simulink model "NetworkOrgignalparametrs3Copter"  (R2020a)
settings: Solver=FixedStepAuto  StartTime=0.0  StopTime=3  FixedStep=0.01  RelTol=1e-3
values from neighbouring files (symbols this model uses):
  Te = 0.012    [4двигателядообученный.mat]    (also in deepLearning.m; tdeepLearning.m)
  Tm = 0.025    [4двигателядообученный.mat]    (also in deepLearning.m; tdeepLearning.m)
  x1 = 1    [4двигателядообученный.mat]
  x2 = 1    [4двигателядообученный.mat]
  x3 = 1    [4двигателядообученный.mat]
libraries: dspsrcs4 x2, vrlib x1, rllib x1
settings Model: Creator=xreno  LastModifiedBy=xreno

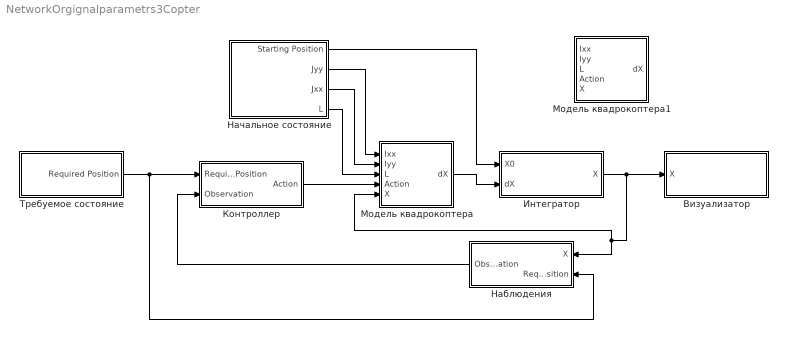
== system NetworkOrgignalparametrs3Copter ==
  Визуализатор : Subsystem
  Интегратор : Subsystem
  Контроллер : Subsystem
  Модель квадрокоптера : Subsystem
  Модель квадрокоптера1 : Subsystem
  Наблюдения : Subsystem
  Начальное состояние : Subsystem
  Требуемое состояние : Subsystem
  wires:
  Начальное состояние/2(Jyy) -> Модель квадрокоптера/1(Ixx)
  Начальное состояние/1(Starting Position) -> Интегратор/1(X0)
  Модель квадрокоптера/1(dX) -> Интегратор/2(dX)
  Требуемое состояние/1(Required Position) -> Наблюдения/2(Required Position), Контроллер/1(Required Position)
  Интегратор/1(X) -> Модель квадрокоптера/5(X), Наблюдения/1(X), Визуализатор/1(X)
  Начальное состояние/3(Jxx) -> Модель квадрокоптера/2(Iyy)
  Наблюдения/1(Observation) -> Контроллер/2(Observation)
  Начальное состояние/4(L) -> Модель квадрокоптера/3(L)
  Контроллер/1(Action) -> Модель квадрокоптера/4(Action)

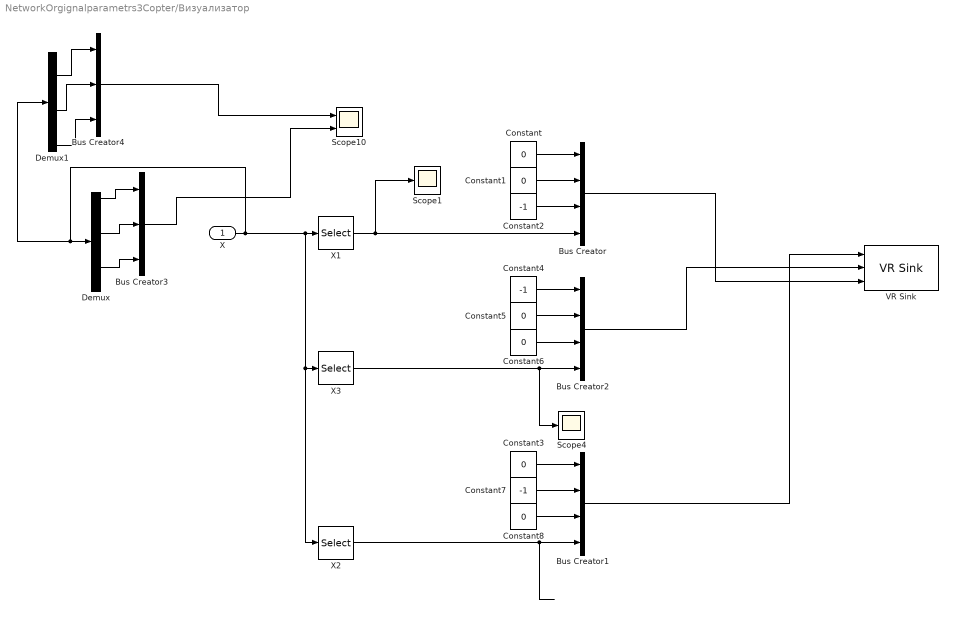
== system NetworkOrgignalparametrs3Copter/Визуализатор ==
  X : Inport
  Bus Creator : BusCreator  Inputs=4
  Bus Creator1 : BusCreator  Inputs=4
  Bus Creator2 : BusCreator  Inputs=4
  Bus Creator3 : BusCreator  Inputs=3
  Bus Creator4 : BusCreator  Inputs=3
  Constant{,1,3,5..6,8} (6 alike) : Constant  Value=0
  Constant2 : Constant  Value=-1
  Constant4 : Constant  Value=-1
  Constant7 : Constant  Value=-1
  Demux : Demux  Outputs=6
  Demux1 : Demux  Outputs=6
  Scope1 : Scope
  Scope10 : Scope  NumInputPorts=2
  Scope4 : Scope
  VR Sink : vrlib/VR Sink  InstantiateOnLoad=on  SampleTime=0.1  ViewEnable=on  RemoteChange=off  RemoteView=off  FieldsWritten=plane1.rotation.4.1.1.double#plane.rotation.4.1.1.double#quadro.rotation.4.1.1.double  WorldFileName=vrml1.wrl  AutoView=off  VideoDimensions=[200 320]  AllowVariableSize=off  FigureProperties="{'Position', 'Name', 'Viewpoint', 'CameraBound', 'CameraDirection', 'CameraPosition', 'CameraUpVector', 'ZoomFactor', 'Antialiasing', 'Headlight', 'Lighting', 'NavPanel', 'Sound', 'StatusBar', 'Stereo3D', 'Stereo3DCameraOffset', 'Stereo3DHIT', 'ToolBar', 'Textures', 'Transparency', 'Triad', 'Wireframe', 'NavZones', 'NavMode', 'NavSpeed', 'CaptureFileFormat', 'CaptureFileName', 'Record2DCompressMethod', 'Record2DCompressQuality', 'Record2D', 'Record2DFileName', 'Record2DFPS'; [1.0000000000000000e+00   7.4199999999999932e+01   1.5360000000000000e+03   6.9880000000000007e+02], '', '', 'on', [2.8420161502207653e-01  -9.0409149145346668e-01   3.1913636129464429e-01], [-2.2963536788759655e+00   7.6675017673078454e+00  -3.2677930566335149e+00], [6.8720478396535467e-01   4.2419952847847997e-01   5.8974939163497742e-01], [1.0000000000000000e+00], 'on', 'on', 'on', 'halfbar', 'on', 'on', 'off', [1.0000000149011612e-01], [0.0000000000000000e+00], 'on', 'on', 'on', 'none', 'off', 'off', 'examine', 'normal', 'tif', '%f_anim_%n.tif', 'auto', [7.5000000000000000e+01], 'on', '%f_anim_%n.avi', 'auto'}"
  X1 : Selector  InputPortWidth=6  IndexOptions=Index vector (dialog)  Indices=[1]  OutputSizes=1
  X2 : Selector  InputPortWidth=6  IndexOptions=Index vector (dialog)  Indices=[5]  OutputSizes=1
  X3 : Selector  InputPortWidth=6  IndexOptions=Index vector (dialog)  Indices=[3]  OutputSizes=1
  wires:
  Constant5/1 -> Bus Creator2/2
  Constant4/1 -> Bus Creator2/1
  Constant1/1 -> Bus Creator/2
  Bus Creator2/1 -> VR Sink/2
  Constant6/1 -> Bus Creator2/3
  Constant2/1 -> Bus Creator/3
  Constant/1 -> Bus Creator/1
  Bus Creator/1 -> VR Sink/3
  X1/1 -> Bus Creator/4, Scope1/1
  X3/1 -> Scope4/1, Bus Creator2/4
  Constant3/1 -> Bus Creator1/1
  X2/1 -> Bus Creator1/4
  Constant7/1 -> Bus Creator1/2
  Constant8/1 -> Bus Creator1/3
  Bus Creator1/1 -> VR Sink/1
  Demux/3 -> Bus Creator3/2
  Demux/5 -> Bus Creator3/3
  Demux/1 -> Bus Creator3/1
  Bus Creator3/1 -> Scope10/2
  X/1 -> Demux1/1, Demux/1, X2/1, X3/1, X1/1
  Demux1/2 -> Bus Creator4/1
  Demux1/4 -> Bus Creator4/2
  Demux1/6 -> Bus Creator4/3
  Bus Creator4/1 -> Scope10/1

== system NetworkOrgignalparametrs3Copter/Интегратор ==
  X0 : Inport
  dX : Inport  Port=2
  Integrator2 : Integrator  InitialConditionSource=external
  X : Outport
  wires:
  X0/1 -> Integrator2/2
  dX/1 -> Integrator2/1
  Integrator2/1 -> X/1

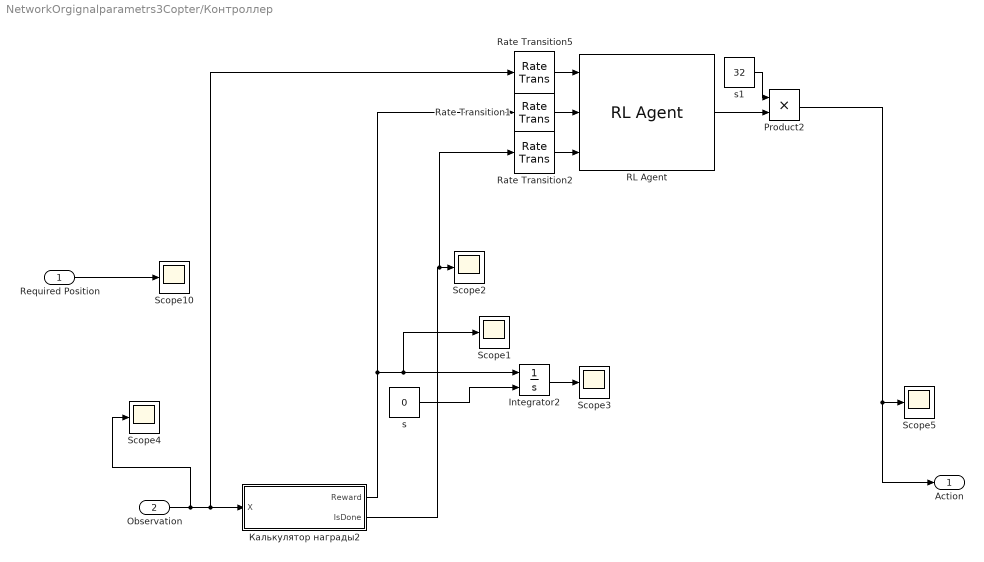
== system NetworkOrgignalparametrs3Copter/Контроллер ==
  Required Position : Inport
  Observation : Inport  Port=2
  Integrator2 : Integrator  InitialConditionSource=external
  Product2 : Product
  RL Agent : rllib/RL Agent  Agent=agent  ProvideReward=on  ProvideIsDone=on  ProvideCumRwd=off  TreatAsDirectFeedthrough=on  CollectLoggedSignals=on  CollectModelStates=on
  Rate Transition1 : RateTransition
  Rate Transition2 : RateTransition
  Rate Transition5 : RateTransition
  Scope{1..5,10} (6 alike) : Scope
  s : Constant  Value=0
  s1 : Constant  Value=32
  Калькулятор награды2 : Subsystem
  Action : Outport
  wires:
  Required Position/1 -> Scope10/1
  Integrator2/1 -> Scope3/1
  s/1 -> Integrator2/2
  Калькулятор награды2/1(Reward) -> Rate Transition1/1, Scope1/1, Integrator2/1
  Калькулятор награды2/2(IsDone) -> Rate Transition2/1, Scope2/1
  Product2/1 -> Action/1, Scope5/1
  Observation/1 -> Scope4/1, Rate Transition5/1, Калькулятор награды2/1(X)
  RL Agent/1 -> Product2/2
  s1/1 -> Product2/1
  Rate Transition5/1 -> RL Agent/1
  Rate Transition1/1 -> RL Agent/2
  Rate Transition2/1 -> RL Agent/3

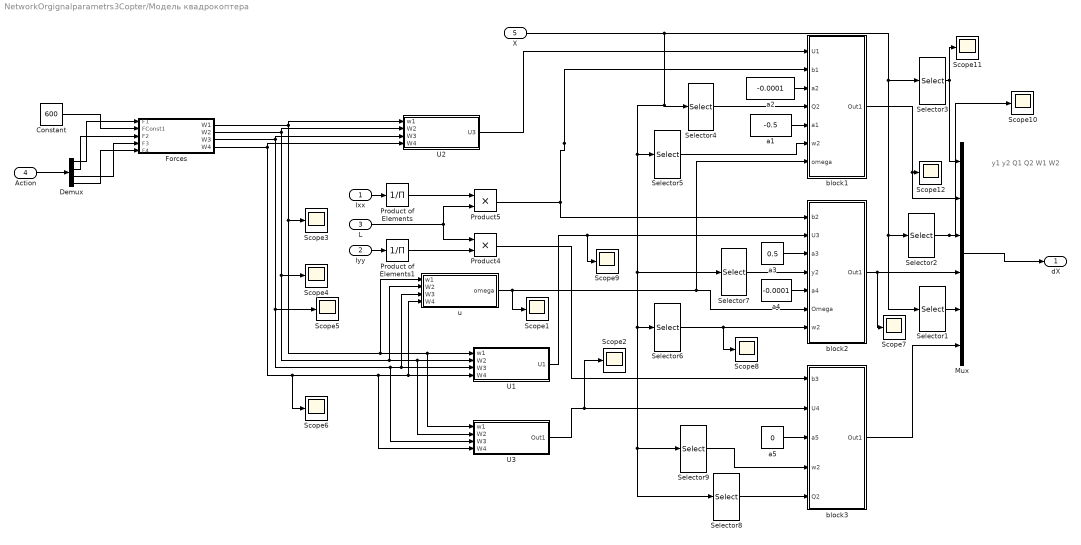
== system NetworkOrgignalparametrs3Copter/Модель квадрокоптера ==
  note: y1
      | y2
      | Q1
      | Q2
      | W1
      | W2
  Ixx : Inport
  Iyy : Inport  Port=2
  L : Inport  Port=3
  Action : Inport  Port=4
  X : Inport  Port=5
  Constant : Constant  Value=600
  Demux : Demux
  Forces : Subsystem
  Mux : Mux  Inputs=6
  Product of Elements : Product  Inputs=/
  Product of Elements1 : Product  Inputs=/
  Product4 : Product
  Product5 : Product
  Scope{1..12} (12 alike) : Scope
  Selector{1,5..6,9} (4 alike) : Selector  InputPortWidth=6  IndexOptions=Index vector (dialog)  Indices=[6]  OutputSizes=1
  Selector2 : Selector  InputPortWidth=6  IndexOptions=Index vector (dialog)  Indices=[4]  OutputSizes=1
  Selector3 : Selector  InputPortWidth=6  IndexOptions=Index vector (dialog)  Indices=[2]  OutputSizes=1
  Selector4 : Selector  InputPortWidth=6  IndexOptions=Index vector (dialog)  Indices=[4]  OutputSizes=1
  Selector7 : Selector  InputPortWidth=6  IndexOptions=Index vector (dialog)  Indices=[2]  OutputSizes=1
  Selector8 : Selector  InputPortWidth=6  IndexOptions=Index vector (dialog)  Indices=[4]  OutputSizes=1
  U1 : Subsystem
  U2 : Subsystem
  U3 : Subsystem
  a1 : Constant  Value=-0.5
  a2 : Constant  Value=-0.0001
  a3 : Constant  Value=0.5
  a4 : Constant  Value=-0.0001
  a5 : Constant  Value=0
  block1 : Subsystem
  block2 : Subsystem
  block3 : Subsystem
  u : Subsystem
  dX : Outport
  wires:
  X/1 -> Selector7/1, Selector8/1, Selector9/1, Selector6/1, Selector5/1, Selector4/1, Selector1/1, Selector2/1, Selector3/1
  Action/1 -> Demux/1
  Mux/1 -> dX/1
  Forces/2(W2) -> U2/2(W2), Scope4/1, u/2(W2), U1/2(W2), U3/2(W2)
  Forces/4(W4) -> U2/4(W4), Scope6/1, U3/4(W4), u/4(W4), U1/4(W4)
  Forces/3(W3) -> U2/3(W3), U3/3(W3), u/3(W3), U1/3(W3), Scope5/1
  U2/1(U3) -> block1/1(U1)
  Product5/1 -> block1/2(b1), block2/1(b2)
  U1/1(U1) -> Scope9/1, block2/2(U3)
  Product of Elements/1 -> Product5/1
  Product of Elements1/1 -> Product4/2
  Product4/1 -> block3/1(b3)
  L/1 -> Product4/1, Product5/2
  Iyy/1 -> Product of Elements1/1
  Ixx/1 -> Product of Elements/1
  Forces/1(W1) -> U2/1(w1), u/1(w1), U1/1(w1), U3/1(w1), Scope3/1
  block1/1(Out1) -> Scope12/1, Mux/2
  block2/1(Out1) -> Scope7/1, Mux/4
  block3/1(Out1) -> Mux/6
  Selector3/1 -> Scope11/1, Mux/1
  Selector2/1 -> Scope10/1, Mux/3
  Selector1/1 -> Mux/5
  u/1(omega) -> Scope1/1, block2/6(Omega), block1/7(omega)
  a3/1 -> block2/3(a3)
  a1/1 -> block1/5(a1)
  a2/1 -> block1/3(a2)
  a4/1 -> block2/5(a4)
  a5/1 -> block3/3(a5)
  U3/1(Out1) -> Scope2/1, block3/2(U4)
  Selector4/1 -> block1/4(Q2)
  Selector5/1 -> block1/6(w2)
  Selector6/1 -> Scope8/1, block2/7(w2)
  Selector7/1 -> block2/4(y2)
  Selector8/1 -> block3/5(Q2)
  Selector9/1 -> block3/4(w2)
  Demux/1 -> Forces/1(F1)
  Constant/1 -> Forces/2(FConst1)
  Demux/2 -> Forces/3(F2)
  Demux/3 -> Forces/4(F3)
  Demux/4 -> Forces/5(F4)

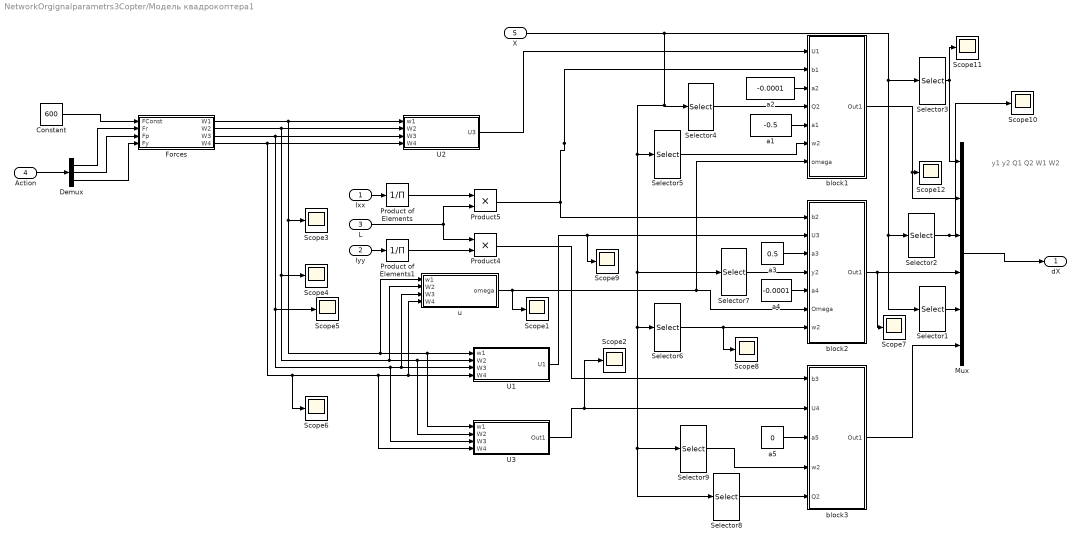
== system NetworkOrgignalparametrs3Copter/Модель квадрокоптера1 ==
  note: y1
      | y2
      | Q1
      | Q2
      | W1
      | W2
  Ixx : Inport
  Iyy : Inport  Port=2
  L : Inport  Port=3
  Action : Inport  Port=4
  X : Inport  Port=5
  Constant : Constant  Value=600
  Demux : Demux  Outputs=3
  Forces : Subsystem
  Mux : Mux  Inputs=6
  Product of Elements : Product  Inputs=/
  Product of Elements1 : Product  Inputs=/
  Product4 : Product
  Product5 : Product
  Scope{1..12} (12 alike) : Scope
  Selector{1,5..6,9} (4 alike) : Selector  InputPortWidth=6  IndexOptions=Index vector (dialog)  Indices=[6]  OutputSizes=1
  Selector2 : Selector  InputPortWidth=6  IndexOptions=Index vector (dialog)  Indices=[4]  OutputSizes=1
  Selector3 : Selector  InputPortWidth=6  IndexOptions=Index vector (dialog)  Indices=[2]  OutputSizes=1
  Selector4 : Selector  InputPortWidth=6  IndexOptions=Index vector (dialog)  Indices=[4]  OutputSizes=1
  Selector7 : Selector  InputPortWidth=6  IndexOptions=Index vector (dialog)  Indices=[2]  OutputSizes=1
  Selector8 : Selector  InputPortWidth=6  IndexOptions=Index vector (dialog)  Indices=[4]  OutputSizes=1
  U1 : Subsystem
  U2 : Subsystem
  U3 : Subsystem
  a1 : Constant  Value=-0.5
  a2 : Constant  Value=-0.0001
  a3 : Constant  Value=0.5
  a4 : Constant  Value=-0.0001
  a5 : Constant  Value=0
  block1 : Subsystem
  block2 : Subsystem
  block3 : Subsystem
  u : Subsystem
  dX : Outport
  wires:
  X/1 -> Selector7/1, Selector8/1, Selector9/1, Selector6/1, Selector5/1, Selector4/1, Selector1/1, Selector2/1, Selector3/1
  Action/1 -> Demux/1
  Mux/1 -> dX/1
  Constant/1 -> Forces/1(FConst)
  Forces/2(W2) -> U2/2(W2), Scope4/1, u/2(W2), U1/2(W2), U3/2(W2)
  Forces/4(W4) -> U2/4(W4), Scope6/1, U3/4(W4), u/4(W4), U1/4(W4)
  Forces/3(W3) -> U2/3(W3), U3/3(W3), u/3(W3), U1/3(W3), Scope5/1
  U2/1(U3) -> block1/1(U1)
  Product5/1 -> block1/2(b1), block2/1(b2)
  U1/1(U1) -> Scope9/1, block2/2(U3)
  Product of Elements/1 -> Product5/1
  Product of Elements1/1 -> Product4/2
  Product4/1 -> block3/1(b3)
  L/1 -> Product4/1, Product5/2
  Iyy/1 -> Product of Elements1/1
  Ixx/1 -> Product of Elements/1
  Forces/1(W1) -> U2/1(w1), u/1(w1), U1/1(w1), U3/1(w1), Scope3/1
  Demux/1 -> Forces/2(Fr)
  Demux/2 -> Forces/3(Fp)
  block1/1(Out1) -> Scope12/1, Mux/2
  block2/1(Out1) -> Scope7/1, Mux/4
  block3/1(Out1) -> Mux/6
  Selector3/1 -> Scope11/1, Mux/1
  Selector2/1 -> Scope10/1, Mux/3
  Selector1/1 -> Mux/5
  u/1(omega) -> Scope1/1, block2/6(Omega), block1/7(omega)
  a3/1 -> block2/3(a3)
  a1/1 -> block1/5(a1)
  a2/1 -> block1/3(a2)
  a4/1 -> block2/5(a4)
  a5/1 -> block3/3(a5)
  U3/1(Out1) -> Scope2/1, block3/2(U4)
  Selector4/1 -> block1/4(Q2)
  Selector5/1 -> block1/6(w2)
  Selector6/1 -> Scope8/1, block2/7(w2)
  Selector7/1 -> block2/4(y2)
  Selector8/1 -> block3/5(Q2)
  Selector9/1 -> block3/4(w2)
  Demux/3 -> Forces/4(Fy)

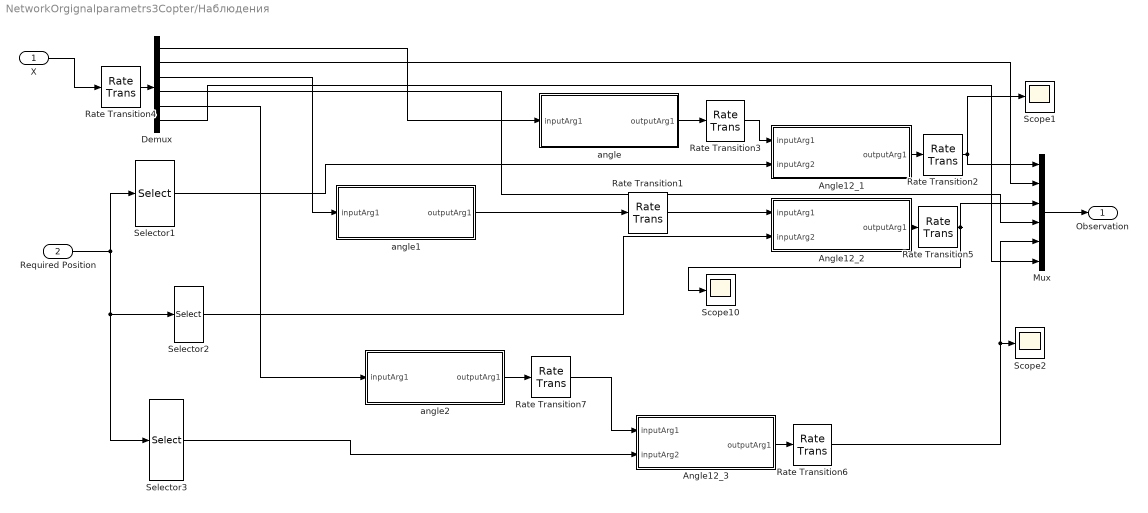
== system NetworkOrgignalparametrs3Copter/Наблюдения ==
  X : Inport
  Required Position : Inport  Port=2
  Angle12_1 : MATLAB Function  TreatAsAtomicUnit=on
  Angle12_2 : MATLAB Function  TreatAsAtomicUnit=on
  Angle12_3 : MATLAB Function  TreatAsAtomicUnit=on
  Demux : Demux  Outputs=6
  Mux : Mux  Inputs=6
  Rate Transition{1..7} (7 alike) : RateTransition
  Scope1 : Scope
  Scope10 : Scope
  Scope2 : Scope
  Selector1 : Selector  InputPortWidth=6  IndexOptions=Index vector (dialog)  Indices=[1]  OutputSizes=1
  Selector2 : Selector  InputPortWidth=6  IndexOptions=Index vector (dialog)  Indices=[3]  OutputSizes=1
  Selector3 : Selector  InputPortWidth=6  IndexOptions=Index vector (dialog)  Indices=[5]  OutputSizes=1
  angle : MATLAB Function  TreatAsAtomicUnit=on
  angle1 : MATLAB Function  TreatAsAtomicUnit=on
  angle2 : MATLAB Function  TreatAsAtomicUnit=on
  Observation : Outport
  wires:
  Rate Transition5/1 -> Scope10/1, Mux/3
  Rate Transition2/1 -> Mux/1, Scope1/1
  Mux/1 -> Observation/1
  Required Position/1 -> Selector1/1, Selector3/1, Selector2/1
  Selector1/1 -> Angle12_1/2(inputArg2)
  Demux/3 -> angle1/1(inputArg1)
  angle1/1(outputArg1) -> Rate Transition1/1
  Rate Transition3/1 -> Angle12_1/1(inputArg1)
  Demux/2 -> Mux/2
  Demux/4 -> Mux/4
  Selector2/1 -> Angle12_2/2(inputArg2)
  X/1 -> Rate Transition4/1
  Rate Transition6/1 -> Scope2/1, Mux/5
  Rate Transition7/1 -> Angle12_3/1(inputArg1)
  Selector3/1 -> Angle12_3/2(inputArg2)
  Demux/5 -> angle2/1(inputArg1)
  Demux/6 -> Mux/6
  angle/1(outputArg1) -> Rate Transition3/1
  Demux/1 -> angle/1(inputArg1)
  Angle12_1/1(outputArg1) -> Rate Transition2/1
  Rate Transition4/1 -> Demux/1
  Rate Transition1/1 -> Angle12_2/1(inputArg1)
  Angle12_2/1(outputArg1) -> Rate Transition5/1
  Angle12_3/1(outputArg1) -> Rate Transition6/1
  angle2/1(outputArg1) -> Rate Transition7/1

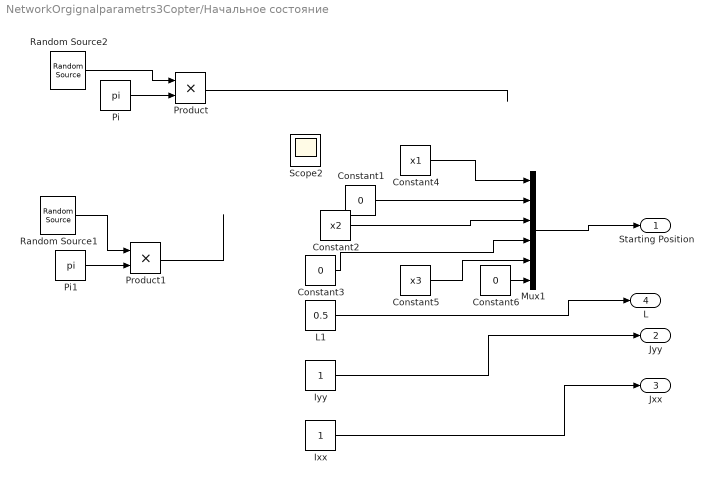
== system NetworkOrgignalparametrs3Copter/Начальное состояние ==
  Constant1 : Constant  Value=0
  Constant2 : Constant  Value=x2
  Constant3 : Constant  Value=0
  Constant4 : Constant  Value=x1
  Constant5 : Constant  Value=x3
  Constant6 : Constant  Value=0
  Ixx : Constant
  Iyy : Constant
  L1 : Constant  Value=0.5
  Mux1 : Mux  Inputs=6
  Pi : Constant  Value=pi  OutDataTypeStr=Inherit: Inherit via back propagation
  Pi1 : Constant  Value=pi  OutDataTypeStr=Inherit: Inherit via back propagation
  Product : Product
  Product1 : Product
  Random Source1 : dspsrcs4/Random Source  SrcType=Uniform  NormMethod=Ziggurat  CltLength=12  MinVal=-1  MaxVal=1  MeanVal=0  VarVal=1  RepMode=Not repeatable  rawSeed=1  IsInherit=off  SampMode=Discrete  SampTime=1  SampFrame=1  DataType=Double  OutComplex=Real  OutputFrames=off
  Random Source2 : dspsrcs4/Random Source  SrcType=Uniform  NormMethod=Ziggurat  CltLength=12  MinVal=-1  MaxVal=1  MeanVal=0  VarVal=1  RepMode=Not repeatable  rawSeed=1  IsInherit=off  SampMode=Discrete  SampTime=1  SampFrame=1  DataType=Double  OutComplex=Real  OutputFrames=off
  Scope2 : Scope
  Starting Position : Outport
  Jyy : Outport  Port=2
  Jxx : Outport  Port=3
  L : Outport  Port=4
  wires:
  Constant1/1 -> Mux1/2
  Mux1/1 -> Starting Position/1
  Constant3/1 -> Mux1/4
  Ixx/1 -> Jxx/1
  Iyy/1 -> Jyy/1
  L1/1 -> L/1
  Pi/1 -> Product/2
  Random Source2/1 -> Product/1
  Random Source1/1 -> Product1/1
  Pi1/1 -> Product1/2
  Product1/1 -> ?
  Product/1 -> ?
  Constant2/1 -> Mux1/3
  Constant4/1 -> Mux1/1
  Constant5/1 -> Mux1/5
  Constant6/1 -> Mux1/6

== system NetworkOrgignalparametrs3Copter/Требуемое состояние ==
  Constant{,1..5} (6 alike) : Constant  Value=0
  Mux1 : Mux  Inputs=6
  Required Position : Outport
  wires:
  Constant/1 -> Mux1/1
  Constant3/1 -> Mux1/4
  Constant1/1 -> Mux1/2
  Mux1/1 -> Required Position/1
  Constant2/1 -> Mux1/3
  Constant4/1 -> Mux1/5
  Constant5/1 -> Mux1/6

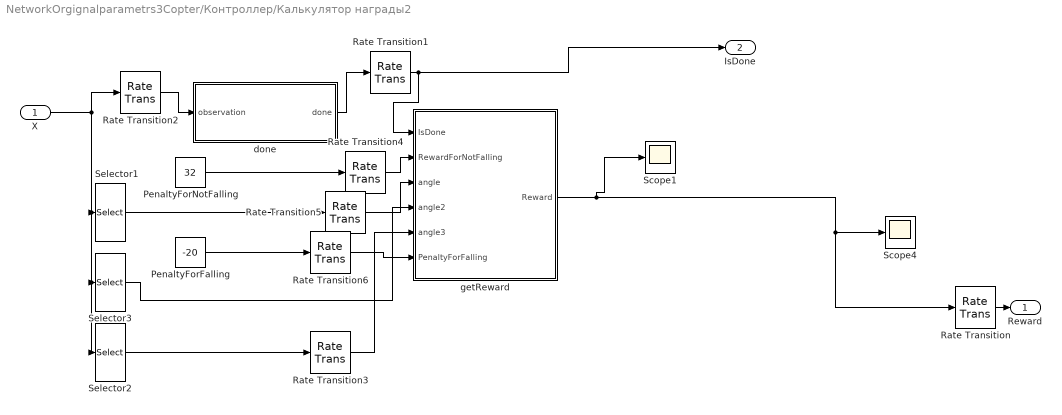
== system NetworkOrgignalparametrs3Copter/Контроллер/Калькулятор награды2 ==
  X : Inport
  PenaltyForFalling : Constant  Value=-20
  PenaltyForNotFalling : Constant  Value=32
  Rate Transition{,1..6} (7 alike) : RateTransition
  Scope1 : Scope
  Scope4 : Scope
  Selector1 : Selector  InputPortWidth=6  IndexOptions=Index vector (dialog)  Indices=[1]  OutputSizes=1
  Selector2 : Selector  InputPortWidth=6  IndexOptions=Index vector (dialog)  Indices=[5]  OutputSizes=1
  Selector3 : Selector  InputPortWidth=6  IndexOptions=Index vector (dialog)  Indices=[3]  OutputSizes=1
  done : MATLAB Function  TreatAsAtomicUnit=on
  getReward : MATLAB Function  TreatAsAtomicUnit=on
  Reward : Outport
  IsDone : Outport  Port=2
  wires:
  X/1 -> Rate Transition2/1, Selector2/1, Selector3/1, Selector1/1
  done/1(done) -> Rate Transition1/1
  PenaltyForFalling/1 -> Rate Transition6/1
  PenaltyForNotFalling/1 -> Rate Transition4/1
  Selector1/1 -> Rate Transition5/1
  getReward/1(Reward) -> Scope4/1, Rate Transition/1, Scope1/1
  Rate Transition/1 -> Reward/1
  Rate Transition2/1 -> done/1(observation)
  Rate Transition1/1 -> getReward/1(IsDone), IsDone/1
  Rate Transition4/1 -> getReward/2(RewardForNotFalling)
  Rate Transition5/1 -> getReward/3(angle)
  Rate Transition6/1 -> getReward/6(PenaltyForFalling)
  Selector3/1 -> getReward/4(angle2)
  Selector2/1 -> Rate Transition3/1
  Rate Transition3/1 -> getReward/5(angle3)

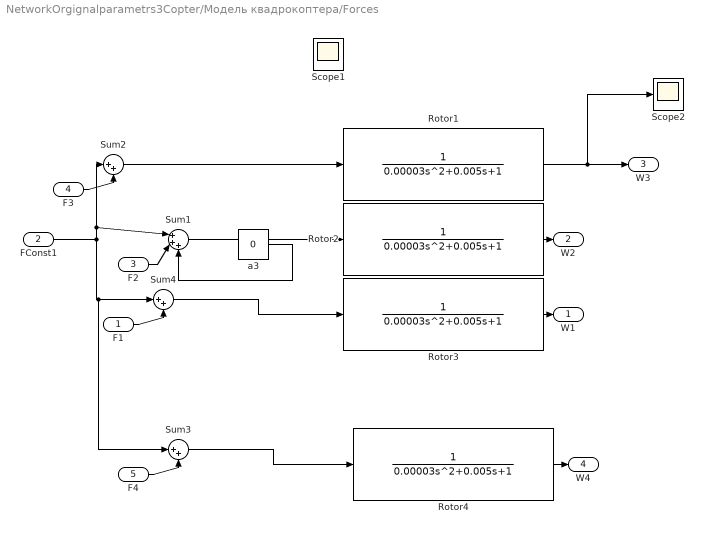
== system NetworkOrgignalparametrs3Copter/Модель квадрокоптера/Forces ==
  F1 : Inport
  FConst1 : Inport  Port=2
  F2 : Inport  Port=3
  F3 : Inport  Port=4
  F4 : Inport  Port=5
  Rotor{1..4} (4 alike) : TransferFcn  Denominator=[0.00003 0.005 1]
  Scope1 : Scope
  Scope2 : Scope
  Sum1 : Sum  Inputs=|+++
  Sum2 : Sum  Inputs=|++
  Sum3 : Sum  Inputs=|++
  Sum4 : Sum  Inputs=|++
  a3 : Constant  Value=0
  W1 : Outport
  W2 : Outport  Port=2
  W3 : Outport  Port=3
  W4 : Outport  Port=4
  wires:
  Rotor1/1 -> Scope2/1, W3/1
  Rotor2/1 -> W2/1
  Rotor3/1 -> W1/1
  Rotor4/1 -> W4/1
  Sum4/1 -> Rotor3/1
  F1/1 -> Sum4/2
  F2/1 -> Sum1/2
  Sum1/1 -> Rotor2/1
  F3/1 -> Sum2/2
  Sum2/1 -> Rotor1/1
  Sum3/1 -> Rotor4/1
  FConst1/1 -> Sum2/1, Sum1/1, Sum3/1, Sum4/1
  F4/1 -> Sum3/2
  a3/1 -> Sum1/3

== system NetworkOrgignalparametrs3Copter/Модель квадрокоптера/U1 ==
  w1 : Inport
  W2 : Inport  Port=2
  W3 : Inport  Port=3
  W4 : Inport  Port=4
  Add : Sum  Inputs=++--
  Product{,1..4} (5 alike) : Product
  b : Constant  Value=0.001
  U1 : Outport
  wires:
  Add/1 -> Product4/2
  W4/1 -> Product3/2, Product3/1
  Product2/1 -> Add/3
  Product/1 -> Add/1
  w1/1 -> Product/2, Product/1
  Product1/1 -> Add/2
  W2/1 -> Product1/2, Product1/1
  W3/1 -> Product2/2, Product2/1
  Product3/1 -> Add/4
  b/1 -> Product4/1
  Product4/1 -> U1/1

== system NetworkOrgignalparametrs3Copter/Модель квадрокоптера/U2 ==
  w1 : Inport
  W2 : Inport  Port=2
  W3 : Inport  Port=3
  W4 : Inport  Port=4
  Add : Sum  Inputs=+-+-
  Product{,1..4} (5 alike) : Product
  b : Constant  Value=0.001
  U3 : Outport
  wires:
  w1/1 -> Product/2, Product/1
  W2/1 -> Product1/2, Product1/1
  W3/1 -> Product2/2, Product2/1
  W4/1 -> Product3/2, Product3/1
  Product/1 -> Add/1
  Product1/1 -> Add/2
  Product2/1 -> Add/3
  Product3/1 -> Add/4
  b/1 -> Product4/1
  Add/1 -> Product4/2
  Product4/1 -> U3/1

== system NetworkOrgignalparametrs3Copter/Модель квадрокоптера/U3 ==
  w1 : Inport
  W2 : Inport  Port=2
  W3 : Inport  Port=3
  W4 : Inport  Port=4
  Add : Sum  Inputs=-++-
  Product{,1..4} (5 alike) : Product
  b1 : Constant  Value=0.0008
  Out1 : Outport
  wires:
  Add/1 -> Product4/2
  W4/1 -> Product3/2, Product3/1
  Product2/1 -> Add/3
  Product/1 -> Add/1
  w1/1 -> Product/2, Product/1
  Product1/1 -> Add/2
  W2/1 -> Product1/2, Product1/1
  W3/1 -> Product2/2, Product2/1
  Product3/1 -> Add/4
  b1/1 -> Product4/1
  Product4/1 -> Out1/1

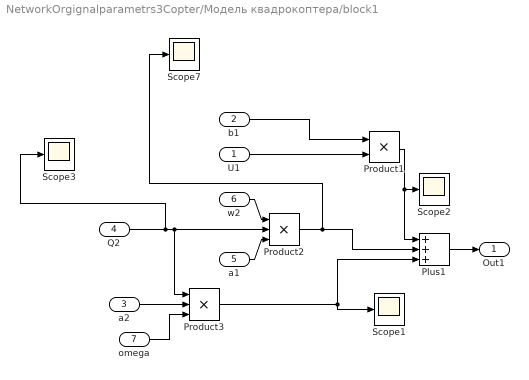
== system NetworkOrgignalparametrs3Copter/Модель квадрокоптера/block1 ==
  U1 : Inport
  b1 : Inport  Port=2
  a2 : Inport  Port=3
  Q2 : Inport  Port=4
  a1 : Inport  Port=5
  w2 : Inport  Port=6
  omega : Inport  Port=7
  Plus1 : Sum  Inputs=+++
  Product1 : Product
  Product2 : Product  Inputs=3
  Product3 : Product  Inputs=3
  Scope{1..3,7} (4 alike) : Scope
  Out1 : Outport
  wires:
  b1/1 -> Product1/1
  U1/1 -> Product1/2
  w2/1 -> Product2/1
  a1/1 -> Product2/3
  Q2/1 -> Scope3/1, Product3/1, Product2/2
  a2/1 -> Product3/2
  omega/1 -> Product3/3
  Product1/1 -> Scope2/1, Plus1/1
  Product2/1 -> Scope7/1, Plus1/2
  Product3/1 -> Plus1/3, Scope1/1
  Plus1/1 -> Out1/1

== system NetworkOrgignalparametrs3Copter/Модель квадрокоптера/block2 ==
  b2 : Inport
  U3 : Inport  Port=2
  a3 : Inport  Port=3
  y2 : Inport  Port=4
  a4 : Inport  Port=5
  Omega : Inport  Port=6
  w2 : Inport  Port=7
  Plus1 : Sum  Inputs=+++
  Product1 : Product
  Product2 : Product  Inputs=3
  Product3 : Product  Inputs=3
  Out1 : Outport
  wires:
  b2/1 -> Product1/1
  U3/1 -> Product1/2
  Omega/1 -> Product2/1
  a4/1 -> Product2/3
  y2/1 -> Product3/1, Product2/2
  a3/1 -> Product3/2
  w2/1 -> Product3/3
  Product1/1 -> Plus1/1
  Product2/1 -> Plus1/2
  Product3/1 -> Plus1/3
  Plus1/1 -> Out1/1

== system NetworkOrgignalparametrs3Copter/Модель квадрокоптера/block3 ==
  b3 : Inport
  U4 : Inport  Port=2
  a5 : Inport  Port=3
  w2 : Inport  Port=4
  Q2 : Inport  Port=5
  Plus1 : Sum  Inputs=-+
  Product1 : Product
  Product3 : Product  Inputs=3
  Out1 : Outport
  wires:
  b3/1 -> Product1/1
  U4/1 -> Product1/2
  a5/1 -> Product3/2
  Product1/1 -> Plus1/1
  Product3/1 -> Plus1/2
  Plus1/1 -> Out1/1
  w2/1 -> Product3/3
  Q2/1 -> Product3/1

== system NetworkOrgignalparametrs3Copter/Модель квадрокоптера/u ==
  w1 : Inport
  W2 : Inport  Port=2
  W3 : Inport  Port=3
  W4 : Inport  Port=4
  Add : Sum  Inputs=+--+
  omega : Outport
  wires:
  w1/1 -> Add/1
  W2/1 -> Add/2
  W3/1 -> Add/3
  W4/1 -> Add/4
  Add/1 -> omega/1

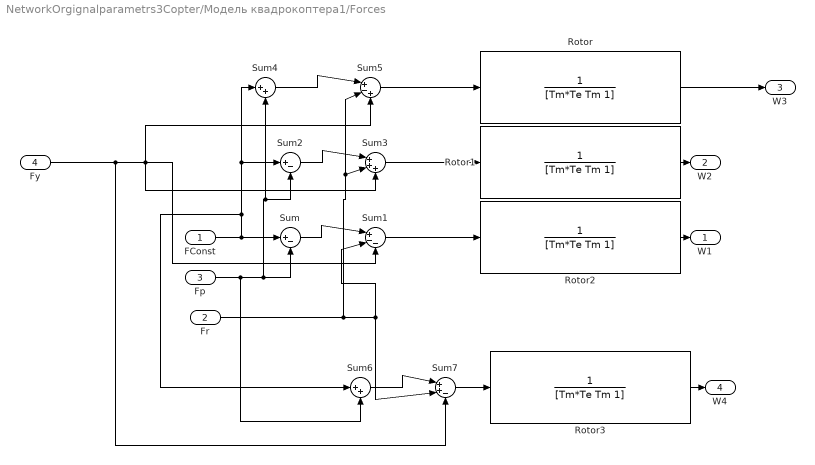
== system NetworkOrgignalparametrs3Copter/Модель квадрокоптера1/Forces ==
  FConst : Inport
  Fr : Inport  Port=2
  Fp : Inport  Port=3
  Fy : Inport  Port=4
  Rotor{,1..3} (4 alike) : TransferFcn  Denominator=[Tm*Te Tm 1]
  Sum : Sum  Inputs=|+-
  Sum1 : Sum  Inputs=|+--
  Sum2 : Sum  Inputs=|+-
  Sum3 : Sum  Inputs=|+++
  Sum4 : Sum  Inputs=|++
  Sum5 : Sum  Inputs=|+-+
  Sum6 : Sum  Inputs=|++
  Sum7 : Sum  Inputs=|++-
  W1 : Outport
  W2 : Outport  Port=2
  W3 : Outport  Port=3
  W4 : Outport  Port=4
  wires:
  Sum/1 -> Sum1/1
  Fp/1 -> Sum6/2, Sum4/2, Sum2/2, Sum/2
  Fr/1 -> Sum3/2, Sum5/2, Sum1/2, Sum7/2
  Sum2/1 -> Sum3/1
  Sum4/1 -> Sum5/1
  Sum6/1 -> Sum7/1
  FConst/1 -> Sum6/1, Sum4/1, Sum2/1, Sum/1
  Sum5/1 -> Rotor/1
  Sum7/1 -> Rotor3/1
  Sum1/1 -> Rotor2/1
  Sum3/1 -> Rotor1/1
  Fy/1 -> Sum1/3, Sum3/3, Sum5/3, Sum7/3
  Rotor/1 -> W3/1
  Rotor1/1 -> W2/1
  Rotor2/1 -> W1/1
  Rotor3/1 -> W4/1

== system NetworkOrgignalparametrs3Copter/Модель квадрокоптера1/U1 ==
  w1 : Inport
  W2 : Inport  Port=2
  W3 : Inport  Port=3
  W4 : Inport  Port=4
  Add : Sum  Inputs=++--
  Product{,1..4} (5 alike) : Product
  b : Constant  Value=0.001
  U1 : Outport
  wires:
  Add/1 -> Product4/2
  W4/1 -> Product3/2, Product3/1
  Product2/1 -> Add/3
  Product/1 -> Add/1
  w1/1 -> Product/2, Product/1
  Product1/1 -> Add/2
  W2/1 -> Product1/2, Product1/1
  W3/1 -> Product2/2, Product2/1
  Product3/1 -> Add/4
  b/1 -> Product4/1
  Product4/1 -> U1/1

== system NetworkOrgignalparametrs3Copter/Модель квадрокоптера1/U2 ==
  w1 : Inport
  W2 : Inport  Port=2
  W3 : Inport  Port=3
  W4 : Inport  Port=4
  Add : Sum  Inputs=+-+-
  Product{,1..4} (5 alike) : Product
  b : Constant  Value=0.001
  U3 : Outport
  wires:
  w1/1 -> Product/2, Product/1
  W2/1 -> Product1/2, Product1/1
  W3/1 -> Product2/2, Product2/1
  W4/1 -> Product3/2, Product3/1
  Product/1 -> Add/1
  Product1/1 -> Add/2
  Product2/1 -> Add/3
  Product3/1 -> Add/4
  b/1 -> Product4/1
  Add/1 -> Product4/2
  Product4/1 -> U3/1

== system NetworkOrgignalparametrs3Copter/Модель квадрокоптера1/U3 ==
  w1 : Inport
  W2 : Inport  Port=2
  W3 : Inport  Port=3
  W4 : Inport  Port=4
  Add : Sum  Inputs=-++-
  Product{,1..4} (5 alike) : Product
  b1 : Constant  Value=0.0008
  Out1 : Outport
  wires:
  Add/1 -> Product4/2
  W4/1 -> Product3/2, Product3/1
  Product2/1 -> Add/3
  Product/1 -> Add/1
  w1/1 -> Product/2, Product/1
  Product1/1 -> Add/2
  W2/1 -> Product1/2, Product1/1
  W3/1 -> Product2/2, Product2/1
  Product3/1 -> Add/4
  b1/1 -> Product4/1
  Product4/1 -> Out1/1

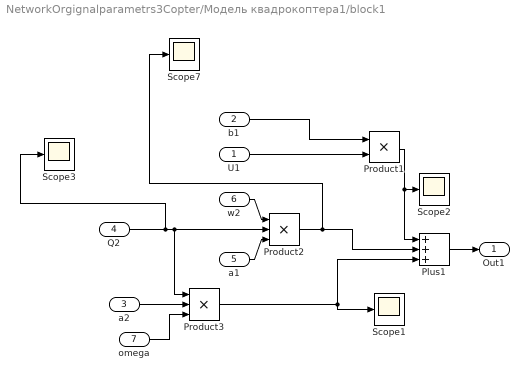
== system NetworkOrgignalparametrs3Copter/Модель квадрокоптера1/block1 ==
  U1 : Inport
  b1 : Inport  Port=2
  a2 : Inport  Port=3
  Q2 : Inport  Port=4
  a1 : Inport  Port=5
  w2 : Inport  Port=6
  omega : Inport  Port=7
  Plus1 : Sum  Inputs=+++
  Product1 : Product
  Product2 : Product  Inputs=3
  Product3 : Product  Inputs=3
  Scope{1..3,7} (4 alike) : Scope
  Out1 : Outport
  wires:
  b1/1 -> Product1/1
  U1/1 -> Product1/2
  w2/1 -> Product2/1
  a1/1 -> Product2/3
  Q2/1 -> Scope3/1, Product3/1, Product2/2
  a2/1 -> Product3/2
  omega/1 -> Product3/3
  Product1/1 -> Scope2/1, Plus1/1
  Product2/1 -> Scope7/1, Plus1/2
  Product3/1 -> Plus1/3, Scope1/1
  Plus1/1 -> Out1/1

== system NetworkOrgignalparametrs3Copter/Модель квадрокоптера1/block2 ==
  b2 : Inport
  U3 : Inport  Port=2
  a3 : Inport  Port=3
  y2 : Inport  Port=4
  a4 : Inport  Port=5
  Omega : Inport  Port=6
  w2 : Inport  Port=7
  Plus1 : Sum  Inputs=+++
  Product1 : Product
  Product2 : Product  Inputs=3
  Product3 : Product  Inputs=3
  Out1 : Outport
  wires:
  b2/1 -> Product1/1
  U3/1 -> Product1/2
  Omega/1 -> Product2/1
  a4/1 -> Product2/3
  y2/1 -> Product3/1, Product2/2
  a3/1 -> Product3/2
  w2/1 -> Product3/3
  Product1/1 -> Plus1/1
  Product2/1 -> Plus1/2
  Product3/1 -> Plus1/3
  Plus1/1 -> Out1/1

== system NetworkOrgignalparametrs3Copter/Модель квадрокоптера1/block3 ==
  b3 : Inport
  U4 : Inport  Port=2
  a5 : Inport  Port=3
  w2 : Inport  Port=4
  Q2 : Inport  Port=5
  Plus1 : Sum  Inputs=-+
  Product1 : Product
  Product3 : Product  Inputs=3
  Out1 : Outport
  wires:
  b3/1 -> Product1/1
  U4/1 -> Product1/2
  a5/1 -> Product3/2
  Product1/1 -> Plus1/1
  Product3/1 -> Plus1/2
  Plus1/1 -> Out1/1
  w2/1 -> Product3/3
  Q2/1 -> Product3/1

== system NetworkOrgignalparametrs3Copter/Модель квадрокоптера1/u ==
  w1 : Inport
  W2 : Inport  Port=2
  W3 : Inport  Port=3
  W4 : Inport  Port=4
  Add : Sum  Inputs=+--+
  omega : Outport
  wires:
  w1/1 -> Add/1
  W2/1 -> Add/2
  W3/1 -> Add/3
  W4/1 -> Add/4
  Add/1 -> omega/1

== matlab function NetworkOrgignalparametrs3Copter/Наблюдения/Angle12_1 ==
  data: outputArg1 output; inputArg1 input; inputArg2 input
function outputArg1 = Angle12(inputArg1,inputArg2)
            %UNTITLED Summary of this function goes here
            % Detailed explanation goes here
            X = inputArg1-inputArg2;
            outputArg1=0;
            
            if (X<-pi)
                outputArg1=X+2*pi;
            end
            if (X>pi)
                outputArg1=X-2*pi;
            end
            if ((X<=pi)&&(X>=-pi))
                outputArg1=X;
            end
            
        end

== matlab function NetworkOrgignalparametrs3Copter/Наблюдения/Angle12_2 ==
  data: outputArg1 output; inputArg1 input; inputArg2 input
function outputArg1 = Angle12(inputArg1,inputArg2)
            %UNTITLED Summary of this function goes here
            % Detailed explanation goes here
            X = inputArg1-inputArg2;
            outputArg1=0;
            
            if (X<-pi)
                outputArg1=X+2*pi;
            end
            if (X>pi)
                outputArg1=X-2*pi;
            end
            if ((X<=pi)&&(X>=-pi))
                outputArg1=X;
            end
            
        end

== matlab function NetworkOrgignalparametrs3Copter/Наблюдения/angle ==
  data: outputArg1 output; inputArg1 input
        function outputArg1 = angle(inputArg1)
            %ANGLE Summary of this function goes here
            % Detailed explanation goes here
            outputArg1=0;
            outputArg1=inputArg1;
            if(inputArg1<0)
                outputArg1 = pi*2+inputArg1;
            end
            if(inputArg1>2*pi)
                outputArg1 = -pi*2+inputArg1;
            end
            
        end

== matlab function NetworkOrgignalparametrs3Copter/Наблюдения/angle1 ==
  data: outputArg1 output; inputArg1 input
        function outputArg1 = angle(inputArg1)
            %ANGLE Summary of this function goes here
            % Detailed explanation goes here
            outputArg1 = 0;
            
            outputArg1=inputArg1;
            if(inputArg1<0)
                outputArg1 = pi*2+inputArg1;
            end
            if(inputArg1>2*pi)
                outputArg1 = -pi*2+inputArg1;
            end
            
        end

== matlab function NetworkOrgignalparametrs3Copter/Наблюдения/Angle12_3 ==
  data: outputArg1 output; inputArg1 input; inputArg2 input
function outputArg1 = Angle12(inputArg1,inputArg2)
            %UNTITLED Summary of this function goes here
            % Detailed explanation goes here
            X = inputArg1-inputArg2;
            outputArg1=0;
            
            if (X<-pi)
                outputArg1=X+2*pi;
            end
            if (X>pi)
                outputArg1=X-2*pi;
            end
            if ((X<=pi)&&(X>=-pi))
                outputArg1=X;
            end
            
        end

== matlab function NetworkOrgignalparametrs3Copter/Наблюдения/angle2 ==
  data: outputArg1 output; inputArg1 input
        function outputArg1 = angle(inputArg1)
            %ANGLE Summary of this function goes here
            % Detailed explanation goes here
            outputArg1=0;
            outputArg1=inputArg1;
            if(inputArg1<0)
                outputArg1 = pi*2+inputArg1;
            end
            if(inputArg1>2*pi)
                outputArg1 = -pi*2+inputArg1;
            end
            
        end

== matlab function NetworkOrgignalparametrs3Copter/Контроллер/Калькулятор награды2/done ==
  settings: updateMethod=DISCRETE
  data: observation input; done output
       function done = isDone(observation)
       done = ((abs(observation(2))>5)||(abs(observation(4))>5)||(abs(observation(6))>5));
       end

== matlab function NetworkOrgignalparametrs3Copter/Контроллер/Калькулятор награды2/getReward ==
  data: IsDone input; Reward output; RewardForNotFalling input; angle input; angle2 input; angle3 input; PenaltyForFalling input
       function Reward = getReward(IsDone, RewardForNotFalling, angle, angle2, angle3, PenaltyForFalling )
            if (IsDone ==0)
                

                Reward=RewardForNotFalling/(abs(angle)+abs(angle2)+abs(angle3)+0.001);

                
                   
                    
            else
                Reward = PenaltyForFalling;
            end 
            
        end
